simulink model "rtwdemo_fixpt1"  (Simulink 7.6)
settings: Solver=FixedStepDiscrete  StartTime=0.0  StopTime=1  MaxStep=.1  RelTol=1e-3  SampleTimeConstraint=Specified
libraries: rtwdemowidgets x2
Description:
  | Fixed-Point Code Generation for Simulink(R), Stateflow(R), and Embedded MATLAB(TM)
settings Model: Creator=The MathWorks Inc.  ExtModeAutoUpdateStatusClock=off
settings MATStruct: SampleTime=0.01  Offset=0  Priority=[41.0]
settings DataIOCC: SaveOutput=off  SaveTime=off  SignalLoggingName=sigsOut
settings OptimizationCC: InlineParams=on  InlineInvariantSignals=on  StateBitsets=on  DataBitsets=on  UseTempVars=on  EfficientFloat2IntCast=on  EfficientMapNaN2IntZero=off  BufferReusableBoundary=off
settings DebuggingCC: CheckExecutionContextPreStartOutputMsg=on  CheckExecutionContextRuntimeOutputMsg=on  SolverPrmCheckMsg=none  ParameterOverflowMsg=warning  ParameterPrecisionLossMsg=none  StrictBusMsg=ErrorOnBusTreatedAsVector
settings HardwareCC: ProdIntDivRoundTo=Zero  ProdEndianess=LittleEndian  ProdHWDeviceType=Generic->32-bit Embedded Processor  TargetHWDeviceType=Generic->32-bit Embedded Processor
settings SFSimCC: SimParseCustomCode=off
settings RTWCC: TLCOptions=-p0 -aWarnNonSaturatedBlocks=0  GenerateReport=on  RTWVerbose=off  ProcessScript=grt_make_rtw_hook  LaunchReport=on
settings CodeAppCC: ForceParamTrailComments=on
settings GRTTargetCC: TargetFcnLib=ansi_tfl_tmw.mat

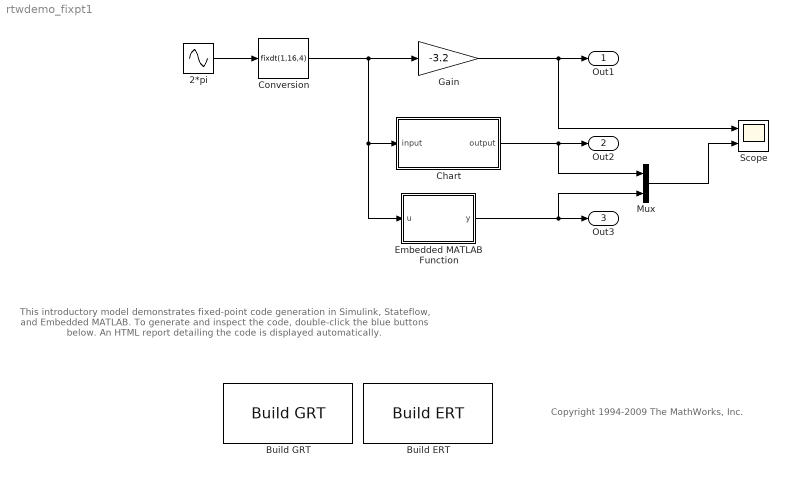
== system rtwdemo_fixpt1 ==
  note: This introductory model demonstrates fixed-point code generation in Simulink, Stateflow,
      | and Embedded MATLAB.  To generate and inspect the code, double-click the blue
      | buttons below.  An HTML report detailing the code is displayed automatically.
  note: Copyright 1994-2009 The MathWorks, Inc.
  2*pi : Sin  SineType=Sample based  Frequency=2*pi  Samples=100  SampleTime=.01
  Build ERT : rtwdemowidgets/Build ERT  SystemSampleTime=-1  attrib_overrides={}
  Build GRT : rtwdemowidgets/Build GRT  SystemSampleTime=-1  attrib_overrides={}
  Chart : Stateflow chart  TreatAsAtomicUnit=on
  Conversion : DataTypeConversion  OutDataTypeStr=fixdt(1,16,4)
  Embedded MATLAB Function : Stateflow chart  TreatAsAtomicUnit=on
  Gain : Gain  Gain=-3.2  ParamDataTypeStr=fixdt(1,16,4)  OutDataTypeStr=fixdt(1,16,4)
  Mux : Mux  Inputs=2
  Scope : Scope  NumInputPorts=2
      settings: TimeRange=1  YMin=-5~-2  YMax=5~4
  Out1 : Outport
  Out2 : Outport  Port=2
  Out3 : Outport  Port=3
  wires:
  2*pi/1 -> Conversion/1
  Gain/1 -> Out1/1, Scope/1
  Chart/1(output) -> Out2/1, Mux/1
  Conversion/1 -> Embedded MATLAB Function/1(u), Chart/1(input), Gain/1
  Embedded MATLAB Function/1(y) -> Out3/1, Mux/2
  Mux/1 -> Scope/2

== stateflow chart Chart ==
  state out = fixout(fixin) [function]
    (default) -> (junction 5)
    (junction 5) -> (junction 6) [order 1] : [fixin>=0.5c]{out = 3.2c*fixin;}
    (junction 5) -> (junction 7) [order 2] : {out = -3.2c*fixin;}
  (default) -> (junction 4) : {output=fixout(input);}
  data: fixin function_input fixdt(1,16,4); out function_output fixdt(1,16,4); input input fixdt(1,16,4); output output fixdt(1,16,4)

== matlab function Embedded MATLAB Function ==
  settings: fimath=fimath('OverFlowMode','Wrap','RoundMode','floor')
  data: u input double; y output fixdt(1,16,4)
function y = fcn(u)
% Simple fixed-point operation without saturation checking. 

f = fimath(u);
c = fi(3.2, f);

if u >= 0.5
    x = u * c;
else
    x = -u * c;
end

% x is a 32 bit fixed point value because it is the result of
% the multiplying two 16 bit values. The fi operation below 
% converts it back to 16 bits.
y = fi(x, 1, 16, 4);
